simulink model "picomotor_model"  (R2014a)
settings: Solver=ode45  StartTime=0.0  StopTime=10.0  RelTol=1e-3
libraries: simulink x1, simulink_extras x1
settings Model: Creator=krish  LastModifiedBy=krish
settings DebuggingCC: SolverPrmCheckMsg=none  IntegerOverflowMsg=none

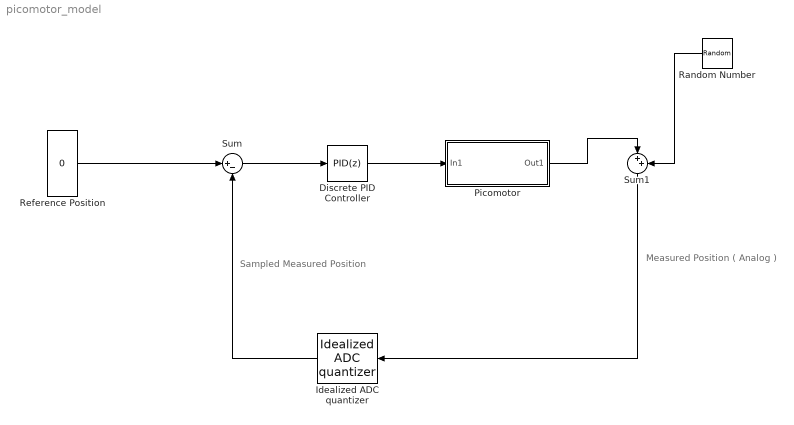
== system picomotor_model ==
  note: Measured
      | Position ( Analog )
  note: Sampled
      | Measured
      | Position
  Discrete PID Controller : simulink/Continuous/PID Controller  Controller=PID  TimeDomain=Discrete-time  SampleTime=1  IntegratorMethod=Forward Euler  FilterMethod=Forward Euler  Form=Parallel  P=1  I=1  D=1  N=100  InitialConditionSource=internal  InitialConditionForIntegrator=0  InitialConditionForFilter=0  ExternalReset=none  IgnoreLimit=on  LimitOutput=off  UpperSaturationLimit=6  LowerSaturationLimit=-6  LinearizeAsGain=off  AntiWindupMode=none  Kb=1  TrackingMode=off  Kt=1  PParamMin=[]  PParamMax=[]  IParamMin=[]  IParamMax=[]  DParamMin=[]  DParamMax=[]  NParamMin=[]  NParamMax=[]  KbParamMin=[]  KbParamMax=[]  KtParamMin=[]  KtParamMax=[]  POutMin=[]  POutMax=[]  IOutMin=[]  IOutMax=[]  DOutMin=[]  DOutMax=[]  NOutMin=[]  NOutMax=[]  KbOutMin=[]  KbOutMax=[]  KtOutMin=[]  KtOutMax=[]  IntegratorOutMin=[]  IntegratorOutMax=[]  FilterOutMin=[]  FilterOutMax=[]  SumOutMin=[]  SumOutMax=[]  SumI1OutMin=[]  SumI1OutMax=[]  SumI2OutMin=[]  SumI2OutMax=[]  SumI3OutMin=[]  SumI3OutMax=[]  SumDOutMin=[]  SumDOutMax=[]  SaturationOutMin=[]  SaturationOutMax=[]  IntegratorContinuousStateAttributes=''  IntegratorStateMustResolveToSignalObject=off  IntegratorRTWStateStorageClass=Auto  FilterContinuousStateAttributes=''  FilterStateMustResolveToSignalObject=off  FilterRTWStateStorageClass=Auto
  Idealized ADC quantizer : simulink_extras/Additional Discrete/Idealized ADC quantizer  NumberOfConverterBits=12  Vmin=0  Vmax=5  OutputDataType=int16  OutputNegativeValues=on
  "Picomotor " : Subsystem
  Random Number : RandomNumber  SampleTime=0.1
  Reference Position : Constant  Value=0
  Sum : Sum  Inputs=|+-
  Sum1 : Sum  Inputs=|++
  wires:
  Idealized ADC quantizer/1 -> Sum/2
  Reference Position/1 -> Sum/1
  Sum/1 -> Discrete PID Controller/1
  Discrete PID Controller/1 -> "Picomotor "/1(In1)
  Sum1/1 -> Idealized ADC quantizer/1
  "Picomotor "/1(Out1) -> Sum1/1
  Random Number/1 -> Sum1/2

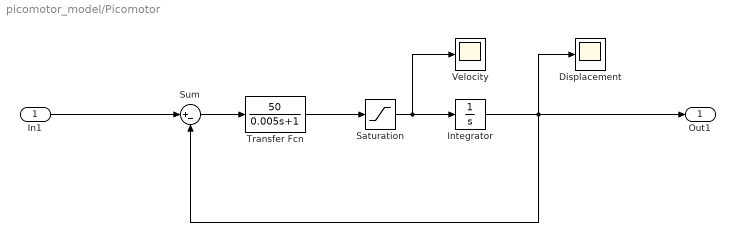
== system picomotor_model/Picomotor  ==
  In1 : Inport  OutMin=-6  OutMax=6
  "Displacement " : Scope
  Integrator : Integrator
  Saturation : Saturate
  Sum : Sum  Inputs=|+-
  Transfer Fcn : TransferFcn  Numerator=[50]  Denominator=[0.005 1]
  Velocity : Scope
      settings: TimeRange=10
  Out1 : Outport
  wires:
  Transfer Fcn/1 -> Saturation/1
  Saturation/1 -> Velocity/1, Integrator/1
  Integrator/1 -> "Displacement "/1, Sum/2, Out1/1
  Sum/1 -> Transfer Fcn/1
  In1/1 -> Sum/1
